simulink model "PID_simulation"  (Simulink 8.5)
settings: Solver=ode113  StartTime=0.0  StopTime=14  RelTol=1e-12  AbsTol=1e-12
undefined symbols (not defined in the file): P, sample_time
settings Model: Creator=Paul_local  LastModifiedBy=User
settings DataIOCC: SaveFormat=StructureWithTime  SignalLoggingSaveFormat=Dataset
settings OptimizationCC: ExpressionDepthLimit=128  EfficientFloat2IntCast=on
settings DebuggingCC: UnderspecifiedInitializationDetection=Simplified  MergeDetectMultiDrivingBlocksExec=error  FcnCallInpInsideContextMsg=EnableAllAsError  StateNameClashWarn=none
settings HardwareCC: ProdBitPerLong=64  ProdBitPerPointer=64  ProdLargestAtomicFloat=Float  ProdIntDivRoundTo=Zero  ProdEndianess=LittleEndian  ProdWordSize=64  ProdHWDeviceType=Intel->x86-64 (Windows64)
settings RTWCC: CheckMdlBeforeBuild=Warning
settings GRTTargetCC: GeneratePreprocessorConditionals=Use local settings  CombineOutputUpdateFcns=on  GRTInterface=off
settings ConfigComp: CovMetricSettings=dw  CovHtmlReporting=on  CovSaveCumulativeToWorkspaceVar=on  CovSaveSingleToWorkspaceVar=on  CovExternalEMLEnable=off

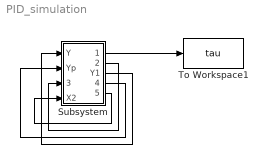
== system PID_simulation ==
  Subsystem : Subsystem
  To Workspace1 : ToWorkspace  VariableName=tau  SaveFormat=Structure With Time  SampleTime=-1
  wires:
  Subsystem/2(Ym1) -> Subsystem/3(Ym)
  Subsystem/5(x21) -> Subsystem/4(X2)
  Subsystem/3(Y1) -> Subsystem/1(Y)
  Subsystem/4(Yp1) -> Subsystem/2(Yp)
  Subsystem/1(tau) -> To Workspace1/1

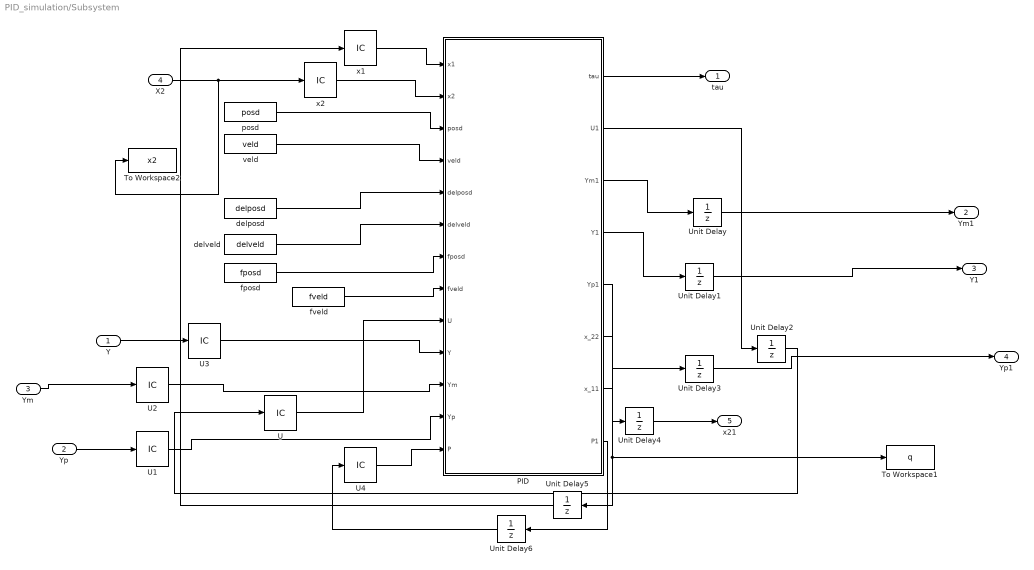
== system PID_simulation/Subsystem ==
  Y : Inport  PortDimensions=[14]
  Yp : Inport  Port=2  PortDimensions=[14]
  Ym : Inport  Port=3  PortDimensions=[14]
  X2 : Inport  Port=4  PortDimensions=[7]
  PID : MATLAB Function  TreatAsAtomicUnit=on
  To Workspace1 : ToWorkspace  VariableName=q  SaveFormat=Structure With Time  SampleTime=-1
  To Workspace2 : ToWorkspace  VariableName=x2  SaveFormat=Structure With Time  SampleTime=-1
  U : InitialCondition  Value=[0 0 0 0 0 0 0]
  U1 : InitialCondition  Value=[-0.1106,-1.9490,-0.0192,3.18400,0.2825,0.0969,-0.2798 0 0 0 0 0 0 0]
  U2 : InitialCondition  Value=[-0.1106,-1.9490,-0.0192,3.18400,0.2825,0.0969,-0.2798 0 0 0 0 0 0 0]
  U3 : InitialCondition  Value=[-0.1106,-1.9490,-0.0192,3.18400,0.2825,0.0969,-0.2798 0 0 0 0 0 0 0]
  U4 : InitialCondition  Value=P
  Unit Delay : UnitDelay  InitialCondition=[-0.1106,-1.9490,-0.0192,3.18400,0.2825,0.0969,-0.2798 0 0 0 0 0 0 0]  SampleTime=sample_time
  Unit Delay1 : UnitDelay  InitialCondition=[-0.1106,-1.9490,-0.0192,3.18400,0.2825,0.0969,-0.2798 0 0 0 0 0 0 0]  SampleTime=sample_time
  Unit Delay2 : UnitDelay  SampleTime=sample_time
  Unit Delay3 : UnitDelay  InitialCondition=[-0.1106,-1.9490,-0.0192,3.18400,0.2825,0.0969,-0.2798 0 0 0 0 0 0 0]  SampleTime=sample_time
  Unit Delay4 : UnitDelay  SampleTime=sample_time
  Unit Delay5 : UnitDelay  InitialCondition=[-0.1106,-1.9490,-0.0192,3.18400,0.2825,0.0969,-0.2798]  SampleTime=sample_time
  Unit Delay6 : UnitDelay  SampleTime=sample_time
  "delposd " : FromWorkspace  VariableName=delposd  SampleTime=sample_time
  delveld : FromWorkspace  VariableName=delveld  SampleTime=sample_time
  "fposd " : FromWorkspace  VariableName=fposd  SampleTime=sample_time
  fveld : FromWorkspace  VariableName=fveld  SampleTime=sample_time
  "posd " : FromWorkspace  VariableName=posd  SampleTime=sample_time
  veld : FromWorkspace  VariableName=veld  SampleTime=sample_time
  x1 : InitialCondition  Value=[-0.1106,-1.9490,-0.192,3.18400,0.2825,0.0969,-0.2798]
  x2 : InitialCondition  Value=[0 0 0 0 0 0 0]
  tau : Outport
  Ym1 : Outport  Port=2  PortDimensions=[14]
  Y1 : Outport  Port=3  PortDimensions=[14]
  Yp1 : Outport  Port=4  PortDimensions=[14]
  x21 : Outport  Port=5  PortDimensions=[7]
  wires:
  x1/1 -> PID/1(x1)
  PID/6(x_22) -> Unit Delay4/1
  "delposd "/1 -> PID/5(delposd)
  veld/1 -> PID/4(veld)
  delveld/1 -> PID/6(delveld)
  Y/1 -> U3/1
  x2/1 -> PID/2(x2)
  U3/1 -> PID/10(Y)
  Ym/1 -> U2/1
  Yp/1 -> U1/1
  "posd "/1 -> PID/3(posd)
  Unit Delay2/1 -> U/1
  PID/2(U1) -> Unit Delay2/1
  U/1 -> PID/9(U)
  U2/1 -> PID/11(Ym)
  PID/3(Ym1) -> Unit Delay/1
  fveld/1 -> PID/8(fveld)
  "fposd "/1 -> PID/7(fposd)
  Unit Delay/1 -> Ym1/1
  PID/7(x_11) -> Unit Delay5/1, To Workspace1/1
  PID/1(tau) -> tau/1
  U1/1 -> PID/12(Yp)
  X2/1 -> To Workspace2/1, x2/1
  PID/4(Y1) -> Unit Delay1/1
  Unit Delay1/1 -> Y1/1
  Unit Delay3/1 -> Yp1/1
  PID/5(Yp1) -> Unit Delay3/1
  Unit Delay5/1 -> x1/1
  Unit Delay4/1 -> x21/1
  U4/1 -> PID/13(P)
  PID/8(P1) -> Unit Delay6/1
  Unit Delay6/1 -> U4/1

== matlab function Subsystem/PID ==
  data: x1 input double; x2 input double; posd input double; tau output double; veld input double; delposd input double; delveld input double; fposd input double; fveld input double; U input double; U1 output double; Ym1 output double; Y1 output double; Yp1 output double; x_22 output double; Y input double; Ym input double; Yp input double; x_11 output double; P input double; P1 output double
%
% gravComp7DOFNum Compute inverse dynamics via recursive Newton-Euler formulation
%
% Recursive Newton-Euler for standard Denavit-Hartenberg notation.
%

% Copyright (C) 1993-2011, by Peter I. Corke
%
% This file originally was part of The Robotics Toolbox for Matlab (RTB).
%
% http://www.petercorke.com

%
% Simplified from rne_dh for 7DOF WAM to compute only torque from gravity by Hans Vorsteveld
% Does not use structures from RTB, only the RNE algorithm
%

function [tau,U1,Ym1,Y1,Yp1,x_22,x_11,P1] = PID(x1,x2,posd,veld,delposd,delveld,fposd,fveld,U,Y,Ym,Yp,P)

%-------------------------------------------------------------------------------------
%   SETUP THE ARM
%-------------------------------------------------------------------------------------    
    n = 14;p = 7; q = 14;
    
 Ts=0.002; 


 
 


yddel=[delposd;delveld];
yd = [posd;veld];
fyd=[fposd;fveld];


 

%initial conditions
%x1 = [-0.11060;-1.949;-0.1920;3.1840;0.2825;0.09690;-0.27980];
%x2 = zeros(7,1);
%U = zeros(7,1);
Ae = 0.9*eye(n);
C= eye(14);
Ce = C;
Iq = eye(q);
Oq = zeros(q);
H = [Iq Oq Oq -Ce*Ae;Iq Oq Oq zeros(q,n);Oq Iq Oq zeros(q,n);zeros(n,q) zeros(n,q) zeros(n,q) Ae];
Ib = zeros(3*q,3*q+n);
for k11 = 1:3*q,Ib(k11,k11) = 1;end
sig = 1e-3;
sigR = sig;
sigQ = 1e-4;%1e-3;
alfa = 1e0;
beta = 1e-2;
p1 = alfa*ones(1,3*q);
p2 = beta*ones(1,n);
pb = [p1 p2];

r1 = 5;
r2 = 50;
r3 = 1.5;
rv = 10;
rbb1 = r1*sig^2*ones(1,q/2);
rbb2 = r2*0.1*sig^2*ones(1,q/2);
rbb12 = [rbb1 rbb2];
rbb = [r3*rbb12 rbb12 rbb12];
 
Rb = 1*diag(rbb);
Q = 0*sigQ^2*eye(n);





 Be = Ts*[zeros(7,7);inv(D(x1))];
    Delyd=fyd-yd;
    Del2yd = Delyd*Delyd';
   
    Gd = [Del2yd Oq Oq zeros(q,n); Oq Oq Oq zeros(q,n); Oq Oq Oq zeros(q,n);zeros(n,q) zeros(n,q) zeros(n,q) Q];
   
    
    
   EE = [Ce*Be;zeros(q,p);zeros(q,p);-Be];
    K = inv(EE'*EE)*EE'*H*P*Ib'*inv(Ib*P*Ib' + Rb);
    PHI = H - EE*K*Ib;
    %if max(abs(eig(PHI))) > 1, disp('max(abs(eig(PHI))) > 1'),tk, pause(1),end
   
    P1 = PHI*P*PHI' + EE*K*Rb*K'*EE' + Gd;
    K1 = K(:,1:q);
    K2 = K(:,q+1:2*q);
    K3 = K(:,2*q+1:3*q);
    
    
      %  E = yd - Y ;
       % Ep = ydfut-Yp ;
        %U = U + K1*Ep + K2*E;
        %Ym = Y;
        %Y = Yp;
         %x_1 = x1 ;
       
         %x_11 = x_1; %Since at t=0, velocity is zero
        %XX2 = zeros(7,1);
        %x_22= (-inv(D(x_1))*(transpose(G(x_1)))+ inv(D(x_1))*U)*Ts + XX2 ;
        %Yp = [x_11' x_22']';
       
    
        Em = yddel - Ym ;
        E = yd - Y ;
        Ep = fyd-Yp ;
        U1 = U + K1*Ep + K2*E + K3*Em;
        Ym1 = Y;
        Y1 = Yp;
        
       
        
        
         
       Ts=0.002;   
        % In experimental work you do not add noise instead you only use measurement of position
        x_11 =  x2*Ts + x1; % Here we are estimating position using the extimate of x2 and measurement of x1 at present time
        
        %XX2 = (x_11-x_1)/Ts; 
        %XX2 = (x1-x1d)/Ts; 
        
        %x_22= (-inv(D(pos_meas))*((G(pos_meas)))+ inv(D(pos_meas))*U)*Ts + XX2 ;
        x3=(-inv(D(x1))*((G(x1)))+ inv(D(x1))*U1);
       x_22=  x2 + Ts*x3;
        
        Yp1 = [x_11' x_22']';
       
        tau=U1;
        
        
        
        
        
    
   
end 

function G = G(q)

DH_a = [0 0 0.045 -0.045 0 0 0];
    DH_d = [0 0 .55 0 0.3 0 0.061];
    DH_alpha = [-pi/2 pi/2 -pi/2 pi/2 -pi/2 pi/2 0];
 
    m = [10.7676 3.87 1.8022 2.4 0.1237 0.4979886 0.07548270];
    
    com = zeros(3,7);
    com(:,1) = [-0.00443422; 0.12189039; -0.00066489];
    com(:,2) = [-0.00236983; 0.03105614; 0.01542114 ];
    com(:,3) = [-0.03825858; 0.20750770; 0.00003309];
    com(:,4) = [ 0.00498512;-0.00022942;0.13271662 ];
    com(:,5) = [0.00008921;0.00511217;0.00435824];
    com(:,6) = [-0.00012262;-0.01703194;0.02468336];
    com(:,7) = [-0.00007974;0.00016313;-0.00323552 ];
     
    
    T = zeros(4,4,7);
     
for j=1:7,
        a = DH_a(j);
        d = DH_d(j);
        alpha = DH_alpha(j);
        T(:,:,j) = getTransformDH(a, d, alpha, q(j));
end 
comstar = zeros(4,7);
    comstar(:,1) = [com(:,1);1];
    comstar(:,2) = [com(:,2);1];
    comstar(:,3) = [com(:,3);1];
    comstar(:,4) = [com(:,4);1];
    comstar(:,5) = [com(:,5);1];
    comstar(:,6) = [com(:,6);1];
    comstar(:,7) = [ com(:,7);1];
  
    Q=[0,-1,0,0;
     1,0,0,0;
     0,0,0,0;
     0,0,0,0];
   
 gravity=[0,0,-9.81,0];
 G=zeros(7,1);
 
   G(1)= -m(1)*gravity*Q*T(:,:,1)*comstar(:,1)-m(2)*gravity*Q*T(:,:,1)*T(:,:,2)*comstar(:,2)-m(3)*gravity*Q*T(:,:,1)*T(:,:,2)*T(:,:,3)*comstar(:,3)-m(4)*gravity*Q*T(:,:,1)*T(:,:,2)*T(:,:,3)*T(:,:,4)*comstar(:,4)-m(5)*gravity*Q*T(:,:,1)*T(:,:,2)*T(:,:,3)*T(:,:,4)*T(:,:,5)*comstar(:,5)-m(6)*gravity*Q*T(:,:,1)*T(:,:,2)*T(:,:,3)*T(:,:,4)*T(:,:,5)*T(:,:,6)*comstar(:,6)-m(7)*gravity*Q*T(:,:,1)*T(:,:,2)*T(:,:,3)*T(:,:,4)*T(:,:,5)*T(:,:,6)*T(:,:,7)*comstar(:,7);   
   G(2)= -m(2)*gravity*T(:,:,1)*Q*T(:,:,2)*comstar(:,2)-m(3)*gravity*T(:,:,1)*Q*T(:,:,2)*T(:,:,3)*comstar(:,3)-m(4)*gravity*T(:,:,1)*Q*T(:,:,2)*T(:,:,3)*T(:,:,4)*comstar(:,4)-m(5)*gravity*T(:,:,1)*Q*T(:,:,2)*T(:,:,3)*T(:,:,4)*T(:,:,5)*comstar(:,5)-m(6)*gravity*T(:,:,1)*Q*T(:,:,2)*T(:,:,3)*T(:,:,4)*T(:,:,5)*T(:,:,6)*comstar(:,6)-m(7)*gravity*T(:,:,1)*Q*T(:,:,2)*T(:,:,3)*T(:,:,4)*T(:,:,5)*T(:,:,6)*T(:,:,7)*comstar(:,7);
   G(3)= -m(3)*gravity*T(:,:,1)*T(:,:,2)*Q*T(:,:,3)*comstar(:,3)-m(4)*gravity*T(:,:,1)*T(:,:,2)*Q*T(:,:,3)*T(:,:,4)*comstar(:,4)-m(5)*gravity*T(:,:,1)*T(:,:,2)*Q*T(:,:,3)*T(:,:,4)*T(:,:,5)*comstar(:,5)-m(6)*gravity*T(:,:,1)*T(:,:,2)*Q*T(:,:,3)*T(:,:,4)*T(:,:,5)*T(:,:,6)*comstar(:,6)-m(7)*gravity*T(:,:,1)*T(:,:,2)*Q*T(:,:,3)*T(:,:,4)*T(:,:,5)*T(:,:,6)*T(:,:,7)*comstar(:,7);
   G(4)= -m(4)*gravity*T(:,:,1)*T(:,:,2)*T(:,:,3)*Q*T(:,:,4)*comstar(:,4)-m(5)*gravity*T(:,:,1)*T(:,:,2)*T(:,:,3)*Q*T(:,:,4)*T(:,:,5)*comstar(:,5)-m(6)*gravity*T(:,:,1)*T(:,:,2)*T(:,:,3)*Q*T(:,:,4)*T(:,:,5)*T(:,:,6)*comstar(:,6)-m(7)*gravity*T(:,:,1)*T(:,:,2)*T(:,:,3)*Q*T(:,:,4)*T(:,:,5)*T(:,:,6)*T(:,:,7)*comstar(:,7);
   G(5)= -m(5)*gravity*T(:,:,1)*T(:,:,2)*T(:,:,3)*T(:,:,4)*Q*T(:,:,5)*comstar(:,5)-m(6)*gravity*T(:,:,1)*T(:,:,2)*T(:,:,3)*T(:,:,4)*Q*T(:,:,5)*T(:,:,6)*comstar(:,6)-m(7)*gravity*T(:,:,1)*T(:,:,2)*T(:,:,3)*T(:,:,4)*Q*T(:,:,5)*T(:,:,6)*T(:,:,7)*comstar(:,7);
   G(6)= -m(6)*gravity*T(:,:,1)*T(:,:,2)*T(:,:,3)*T(:,:,4)*T(:,:,5)*Q*T(:,:,6)*comstar(:,6)-m(7)*gravity*T(:,:,1)*T(:,:,2)*T(:,:,3)*T(:,:,4)*T(:,:,5)*Q*T(:,:,6)*T(:,:,7)*comstar(:,7);
   G(7)= -m(7)*gravity*T(:,:,1)*T(:,:,2)*T(:,:,3)*T(:,:,4)*T(:,:,5)*T(:,:,6)*Q*T(:,:,7)*comstar(:,7);
   
end 
function bq = bq(qd)
 
 
 
s=20;
bc = [2.516; 2.581; 2.038; 0.956; 0.323; 0.315; 0.066];
B =  [1.142; 0.946; 0.309; 0.255; 0.025; 0.039; 0.004];
 
bq = bc.*atan(s*qd)*2/pi+B.*qd;
end 

function D =D(q)
DH_a = [0 0 0.045 -0.045 0 0 0];
    DH_d = [0 0 .55 0 0.3 0 0.061];
    DH_alpha = [-pi/2 pi/2 -pi/2 pi/2 -pi/2 pi/2 0];
 
    m = [10.7676 3.87 1.8022 2.4 0.1237 0.4179886 0.07548270];
    
     
    
    com = zeros(3,7);
   com(:,1) = [-0.00443422; 0.12189039; -0.00066489];
    com(:,2) = [-0.00236983; 0.03105614; 0.01542114 ];
    com(:,3) = [-0.03825858; 0.20750770; 0.00003309];
    com(:,4) = [ 0.00498512;-0.00022942;0.13271662 ];
    com(:,5) = [0.00008921;0.00511217;0.00435824];
    com(:,6) = [-0.00012262;-0.01703194;0.02468336];
    com(:,7) = [-0.00007974;0.00016313;-0.00323552 ];
     
    I=zeros(3,3,7);
    
     I(:,:,1) = [ 0.29486350 , -0.00795023 ,-0.00009311;
                 -0.00795023 , 0.11350017 , -0.00018711;
                -0.00009311 , -0.00018711 , 0.25065343];
    I(:,:,2) =[0.02606840 ,-0.00001346 , -0.00011701;
               -0.00001346,  0.01472202 ,0.00003659;
               -0.00011701 , 0.00003659,  0.01934814];
    I(:,:,3) = [0.13671601,  -0.01680434,  0.00000510;
               -0.01680434 , 0.00588354 , -0.00000530;
                0.00000510 , -0.00000530 , 0.13951371];
    I(:,:,4) = [ 0.05719268 , 0.00001467 , 0.00008193;
                 0.00001467 , 0.05716470 , -0.00009417;
                 0.00008193 , -0.00009417 , 0.00300441] ;
    I(:,:,5) =[0.00005587 , 0.00000026,  0.00000000;
               0.00000026 , 0.00007817,  -0.00000083;
               0.00000000 , -0.00000083,  0.00006594];
    I(:,:,6) = [0.00093106,  0.00000148 , -0.00000201;
                0.00000148,  0.00049833 , -0.00022162;
               -0.00000201,  -0.00022162,  0.00057483];
   I(:,:,7) = [0.00003845,  -0.00000019 , 0.00000002;
                -0.00000019, 0.00003878 , -0.00000004;
                0.00000002 ,  -0.00000004, 0.00007408 ];
            T=zeros(4,4,7);
  
             
for j=1:7,
        a = DH_a(j);
        d = DH_d(j);
        alpha = DH_alpha(j);
        T(:,:,j) = getTransformDH(a, d, alpha, q(j));
end 
 
 
 
 
   comstar = zeros(4,7);
    comstar(:,1) = [com(:,1);1];
    comstar(:,2) = [com(:,2);1];
    comstar(:,3) = [com(:,3);1];
    comstar(:,4) = [com(:,4);1];
    comstar(:,5) = [com(:,5);1];
    comstar(:,6) = [com(:,6);1];
    comstar(:,7) = [ com(:,7);1];
  
    Q=[0,-1,0,0;
     1,0,0,0;
     0,0,0,0;
     0,0,0,0];
   
U=zeros(4,4,7,7);
   U(:,:,1,1)= Q*T(:,:,1);
   U(:,:,2,1)= Q*T(:,:,1)*T(:,:,2);
   U(:,:,3,1)= Q*T(:,:,1)*T(:,:,2)*T(:,:,3);
   U(:,:,4,1)= Q*T(:,:,1)*T(:,:,2)*T(:,:,3)*T(:,:,4);
   U(:,:,5,1)= Q*T(:,:,1)*T(:,:,2)*T(:,:,3)*T(:,:,4)*T(:,:,5);
   U(:,:,6,1)= Q*T(:,:,1)*T(:,:,2)*T(:,:,3)*T(:,:,4)*T(:,:,5)*T(:,:,6);
   U(:,:,7,1)= Q*T(:,:,1)*T(:,:,2)*T(:,:,3)*T(:,:,4)*T(:,:,5)*T(:,:,6)*T(:,:,7);
   
   
   U(:,:,2,2)= T(:,:,1)*Q*T(:,:,2);
   U(:,:,3,2)= T(:,:,1)*Q*T(:,:,2)*T(:,:,3);
   U(:,:,4,2)= T(:,:,1)*Q*T(:,:,2)*T(:,:,3)*T(:,:,4);
   U(:,:,5,2)= T(:,:,1)*Q*T(:,:,2)*T(:,:,3)*T(:,:,4)*T(:,:,5);
   U(:,:,6,2)= T(:,:,1)*Q*T(:,:,2)*T(:,:,3)*T(:,:,4)*T(:,:,5)*T(:,:,6);
   U(:,:,7,2)= T(:,:,1)*Q*T(:,:,2)*T(:,:,3)*T(:,:,4)*T(:,:,5)*T(:,:,6)*T(:,:,7);
   
  
   U(:,:,3,3)= T(:,:,1)*T(:,:,2)*Q*T(:,:,3);
   U(:,:,4,3)= T(:,:,1)*T(:,:,2)*Q*T(:,:,3)*T(:,:,4);
   U(:,:,5,3)= T(:,:,1)*T(:,:,2)*Q*T(:,:,3)*T(:,:,4)*T(:,:,5);
   U(:,:,6,3)= T(:,:,1)*T(:,:,2)*Q*T(:,:,3)*T(:,:,4)*T(:,:,5)*T(:,:,6);
   U(:,:,7,3)= T(:,:,1)*T(:,:,2)*Q*T(:,:,3)*T(:,:,4)*T(:,:,5)*T(:,:,6)*T(:,:,7);
   
   U(:,:,4,4)= T(:,:,1)*T(:,:,2)*T(:,:,3)*Q*T(:,:,4);
   U(:,:,5,4)= T(:,:,1)*T(:,:,2)*T(:,:,3)*Q*T(:,:,4)*T(:,:,5);
   U(:,:,6,4)= T(:,:,1)*T(:,:,2)*T(:,:,3)*Q*T(:,:,4)*T(:,:,5)*T(:,:,6);
   U(:,:,7,4)= T(:,:,1)*T(:,:,2)*T(:,:,3)*Q*T(:,:,4)*T(:,:,5)*T(:,:,6)*T(:,:,7);
   
   U(:,:,5,5)= T(:,:,1)*T(:,:,2)*T(:,:,3)*T(:,:,4)*Q*T(:,:,5);
   U(:,:,6,5)= T(:,:,1)*T(:,:,2)*T(:,:,3)*T(:,:,4)*Q*T(:,:,5)*T(:,:,6);
   U(:,:,7,5)= T(:,:,1)*T(:,:,2)*T(:,:,3)*T(:,:,4)*Q*T(:,:,5)*T(:,:,6)*T(:,:,7);
   
   U(:,:,6,6)= T(:,:,1)*T(:,:,2)*T(:,:,3)*T(:,:,4)*T(:,:,5)*Q*T(:,:,6);
   U(:,:,7,6)= T(:,:,1)*T(:,:,2)*T(:,:,3)*T(:,:,4)*T(:,:,5)*Q*T(:,:,6)*T(:,:,7);
   
   U(:,:,7,7)= T(:,:,1)*T(:,:,2)*T(:,:,3)*T(:,:,4)*T(:,:,5)*T(:,:,6)*Q*T(:,:,7);
   
   
   
  
   J=zeros(4,4,7);
 
   
   J(:,:,1)=[0.5*(-I(1,1,1)+I(2,2,1)+I(3,3,1)), I(1,2,1), I(1,3,1), m(1)*com(1,1);
             I(1,2,1) ,0.5*(I(1,1,1)-I(2,2,1)+I(3,3,1)), I(2,3,1), m(1)*com(2,1);
             I(1,3,1), I(2,3,1), 0.5*(I(1,1,1)+I(2,2,1)-I(3,3,1)), m(1)*com(3,1);
              m(1)*com(1,1), m(1)*com(2,1), m(1)*com(3,1), m(1)];
   
    J(:,:,2)=[0.5*(-I(1,1,2)+I(2,2,2)+I(3,3,2)), I(1,2,2), I(1,3,2), m(2)*com(1,2);
             I(1,2,2) ,0.5*(I(1,1,2)-I(2,2,2)+I(3,3,2)), I(2,3,2), m(2)*com(2,2);
             I(1,3,2), I(2,3,2), 0.5*(I(1,1,2)+I(2,2,2)-I(3,3,2)), m(2)*com(3,2);
              m(2)*com(1,2), m(2)*com(2,2), m(2)*com(3,2), m(2)];
   
          
     J(:,:,3)=[0.5*(-I(1,1,3)+I(2,2,3)+I(3,3,3)), I(1,2,3), I(1,3,3), m(3)*com(1,3);
             I(1,2,3) ,0.5*(I(1,1,3)-I(2,2,3)+I(3,3,3)), I(2,3,3), m(3)*com(2,3);
             I(1,3,3), I(2,3,3), 0.5*(I(1,1,3)+I(2,2,3)-I(3,3,3)), m(3)*com(3,3);
              m(3)*com(1,3), m(3)*com(2,3), m(3)*com(3,3), m(3)];      
   
   
    J(:,:,4)=[0.5*(-I(1,1,4)+I(2,2,4)+I(3,3,4)), I(1,2,4), I(1,3,4), m(4)*com(1,4);
             I(1,2,4) ,0.5*(I(1,1,4)-I(2,2,4)+I(3,3,4)), I(2,3,4), m(4)*com(2,4);
             I(1,3,4), I(2,3,4), 0.5*(I(1,1,4)+I(2,2,4)-I(3,3,4)), m(4)*com(3,4);
              m(4)*com(1,4), m(4)*com(2,4), m(4)*com(3,4), m(4)];
   
   
    J(:,:,5)=[0.5*(-I(1,1,5)+I(2,2,5)+I(3,3,5)), I(1,2,5), I(1,3,5), m(5)*com(1,5);
             I(1,2,5) ,0.5*(I(1,1,5)-I(2,2,5)+I(3,3,5)), I(2,3,5), m(5)*com(2,5);
             I(1,3,5), I(2,3,5), 0.5*(I(1,1,5)+I(2,2,5)-I(3,3,5)), m(5)*com(3,5);
              m(5)*com(1,5), m(5)*com(2,5), m(5)*com(3,5), m(5)];
   
   
    J(:,:,6)=[0.5*(-I(1,1,6)+I(2,2,6)+I(3,3,6)), I(1,2,6), I(1,3,6), m(6)*com(1,6);
             I(1,2,6) ,0.5*(I(1,1,6)-I(2,2,6)+I(3,3,6)), I(2,3,6), m(6)*com(2,6);
             I(1,3,6), I(2,3,6), 0.5*(I(1,1,6)+I(2,2,6)-I(3,3,6)), m(6)*com(3,6);
              m(6)*com(1,6), m(6)*com(2,6), m(6)*com(3,6), m(6)];
   
   
    J(:,:,7)=[0.5*(-I(1,1,7)+I(2,2,7)+I(3,3,7)), I(1,2,7), I(1,3,7), m(7)*com(1,7);
             I(1,2,7) ,0.5*(I(1,1,7)-I(2,2,7)+I(3,3,7)), I(2,3,7), m(7)*com(2,7);
             I(1,3,7), I(2,3,7), 0.5*(I(1,1,7)+I(2,2,7)-I(3,3,7)), m(7)*com(3,7);
              m(7)*com(1,7), m(7)*com(2,7), m(7)*com(3,7), m(7)];
   
   D=zeros(7,7);
    D(1,1)= trace(U(:,:,1,1)*J(:,:,1)*transpose(U(:,:,1,1))) + trace(U(:,:,2,1)*J(:,:,2)*transpose(U(:,:,2,1))) + trace(U(:,:,3,1)*J(:,:,3)*transpose(U(:,:,3,1))) + trace(U(:,:,4,1)*J(:,:,4)*transpose(U(:,:,4,1))) + trace(U(:,:,5,1)*J(:,:,5)*transpose(U(:,:,5,1))) + trace(U(:,:,6,1)*J(:,:,6)*transpose(U(:,:,6,1))) + trace(U(:,:,7,1)*J(:,:,7)*transpose(U(:,:,7,1))) ;
    D(1,2)= trace(U(:,:,2,2)*J(:,:,2)*transpose(U(:,:,2,1))) + trace(U(:,:,3,2)*J(:,:,3)*transpose(U(:,:,3,1))) + trace(U(:,:,4,2)*J(:,:,4)*transpose(U(:,:,4,1))) +trace(U(:,:,5,2)*J(:,:,5)*transpose(U(:,:,5,1))) + trace(U(:,:,6,2)*J(:,:,6)*transpose(U(:,:,6,1))) + trace(U(:,:,7,2)*J(:,:,7)*transpose(U(:,:,7,1))); 
    D(1,3)= trace(U(:,:,3,3)*J(:,:,3)*transpose(U(:,:,3,1)))+ trace(U(:,:,4,3)*J(:,:,4)*transpose(U(:,:,4,1)))+ trace(U(:,:,5,3)*J(:,:,5)*transpose(U(:,:,5,1)))+ trace(U(:,:,6,3)*J(:,:,6)*transpose(U(:,:,6,1)))+ trace(U(:,:,7,3)*J(:,:,7)*transpose(U(:,:,7,1))); 
    D(1,4)= trace(U(:,:,4,4)*J(:,:,4)*transpose(U(:,:,4,1)))+ trace(U(:,:,5,4)*J(:,:,5)*transpose(U(:,:,5,1)))+ trace(U(:,:,6,4)*J(:,:,6)*transpose(U(:,:,6,1)))+ trace(U(:,:,7,4)*J(:,:,7)*transpose(U(:,:,7,1)));
    D(1,5)= trace(U(:,:,5,5)*J(:,:,5)*transpose(U(:,:,5,1)))+ trace(U(:,:,6,5)*J(:,:,6)*transpose(U(:,:,6,1)))+ trace(U(:,:,7,5)*J(:,:,7)*transpose(U(:,:,7,1)));
    D(1,6)= trace(U(:,:,6,6)*J(:,:,6)*transpose(U(:,:,6,1)))+ trace(U(:,:,7,6)*J(:,:,7)*transpose(U(:,:,7,1)));
    D(1,7)= trace(U(:,:,7,7)*J(:,:,7)*transpose(U(:,:,7,1)));
    
    D(2,1)= trace(U(:,:,2,1)*J(:,:,2)*transpose(U(:,:,2,2)))+ trace(U(:,:,3,1)*J(:,:,3)*transpose(U(:,:,3,2)))+ trace(U(:,:,4,1)*J(:,:,4)*transpose(U(:,:,4,2)))+ trace(U(:,:,5,1)*J(:,:,5)*transpose(U(:,:,5,2)))+ trace(U(:,:,6,1)*J(:,:,6)*transpose(U(:,:,6,2)))+ trace(U(:,:,7,1)*J(:,:,7)*transpose(U(:,:,7,2)));
    D(2,2)= trace(U(:,:,2,2)*J(:,:,2)*transpose(U(:,:,2,2)))+ trace(U(:,:,3,2)*J(:,:,3)*transpose(U(:,:,3,2)))+ trace(U(:,:,4,2)*J(:,:,4)*transpose(U(:,:,4,2)))+ trace(U(:,:,5,2)*J(:,:,5)*transpose(U(:,:,5,2)))+ trace(U(:,:,6,2)*J(:,:,6)*transpose(U(:,:,6,2)))+ trace(U(:,:,7,2)*J(:,:,7)*transpose(U(:,:,7,2)));
    D(2,3)= trace(U(:,:,3,3)*J(:,:,3)*transpose(U(:,:,3,2)))+ trace(U(:,:,4,3)*J(:,:,4)*transpose(U(:,:,4,2)))+ trace(U(:,:,5,3)*J(:,:,5)*transpose(U(:,:,5,2)))+ trace(U(:,:,6,3)*J(:,:,6)*transpose(U(:,:,6,2)))+ trace(U(:,:,7,3)*J(:,:,7)*transpose(U(:,:,7,2))); 
    D(2,4)= trace(U(:,:,4,4)*J(:,:,4)*transpose(U(:,:,4,2)))+ trace(U(:,:,5,4)*J(:,:,5)*transpose(U(:,:,5,2)))+ trace(U(:,:,6,4)*J(:,:,6)*transpose(U(:,:,6,2)))+ trace(U(:,:,7,4)*J(:,:,7)*transpose(U(:,:,7,2))); 
    D(2,5)= trace(U(:,:,5,5)*J(:,:,5)*transpose(U(:,:,5,2)))+ trace(U(:,:,6,5)*J(:,:,6)*transpose(U(:,:,6,2)))+ trace(U(:,:,7,5)*J(:,:,7)*transpose(U(:,:,7,2)));
    D(2,6)= trace(U(:,:,6,6)*J(:,:,6)*transpose(U(:,:,6,2)))+ trace(U(:,:,7,6)*J(:,:,7)*transpose(U(:,:,7,2))); 
    D(2,7)= trace(U(:,:,7,7)*J(:,:,7)*transpose(U(:,:,7,2)));
  
    D(3,1)= trace(U(:,:,3,1)*J(:,:,3)*transpose(U(:,:,3,3)))+ trace(U(:,:,4,1)*J(:,:,4)*transpose(U(:,:,4,3)))+ trace(U(:,:,5,1)*J(:,:,5)*transpose(U(:,:,5,3)))+ trace(U(:,:,6,1)*J(:,:,6)*transpose(U(:,:,6,3)))+ trace(U(:,:,7,1)*J(:,:,7)*transpose(U(:,:,7,3)));
    D(3,2)= trace(U(:,:,3,2)*J(:,:,3)*transpose(U(:,:,3,3)))+ trace(U(:,:,4,2)*J(:,:,4)*transpose(U(:,:,4,3)))+ trace(U(:,:,5,2)*J(:,:,5)*transpose(U(:,:,5,3)))+ trace(U(:,:,6,2)*J(:,:,6)*transpose(U(:,:,6,3)))+ trace(U(:,:,7,2)*J(:,:,7)*transpose(U(:,:,7,3)));
    D(3,3)= trace(U(:,:,3,3)*J(:,:,3)*transpose(U(:,:,3,3)))+ trace(U(:,:,4,3)*J(:,:,4)*transpose(U(:,:,4,3)))+ trace(U(:,:,5,3)*J(:,:,5)*transpose(U(:,:,5,3)))+ trace(U(:,:,6,3)*J(:,:,6)*transpose(U(:,:,6,3)))+ trace(U(:,:,7,3)*J(:,:,7)*transpose(U(:,:,7,3)));
    D(3,4)= trace(U(:,:,4,4)*J(:,:,4)*transpose(U(:,:,4,3)))+ trace(U(:,:,5,4)*J(:,:,5)*transpose(U(:,:,5,3)))+ trace(U(:,:,6,4)*J(:,:,6)*transpose(U(:,:,6,3)))+ trace(U(:,:,7,4)*J(:,:,7)*transpose(U(:,:,7,3)));
    D(3,5)= trace(U(:,:,5,5)*J(:,:,5)*transpose(U(:,:,5,3)))+ trace(U(:,:,6,5)*J(:,:,6)*transpose(U(:,:,6,3)))+ trace(U(:,:,7,5)*J(:,:,7)*transpose(U(:,:,7,3)));
    D(3,6)= trace(U(:,:,6,6)*J(:,:,6)*transpose(U(:,:,6,3)))+ trace(U(:,:,7,6)*J(:,:,7)*transpose(U(:,:,7,3)));
    D(3,7)= trace(U(:,:,7,7)*J(:,:,7)*transpose(U(:,:,7,3)));
     
     
    D(4,1)= trace(U(:,:,4,1)*J(:,:,4)*transpose(U(:,:,4,4)))+ trace(U(:,:,5,1)*J(:,:,5)*transpose(U(:,:,5,4)))+ trace(U(:,:,6,1)*J(:,:,6)*transpose(U(:,:,6,4)))+ trace(U(:,:,7,1)*J(:,:,7)*transpose(U(:,:,7,4))); 
    D(4,2)= trace(U(:,:,4,2)*J(:,:,4)*transpose(U(:,:,4,4)))+ trace(U(:,:,5,2)*J(:,:,5)*transpose(U(:,:,5,4)))+ trace(U(:,:,6,2)*J(:,:,6)*transpose(U(:,:,6,4)))+ trace(U(:,:,7,2)*J(:,:,7)*transpose(U(:,:,7,4))); 
    D(4,3)= trace(U(:,:,4,3)*J(:,:,4)*transpose(U(:,:,4,4)))+ trace(U(:,:,5,3)*J(:,:,5)*transpose(U(:,:,5,4)))+ trace(U(:,:,6,3)*J(:,:,6)*transpose(U(:,:,6,4)))+ trace(U(:,:,7,3)*J(:,:,7)*transpose(U(:,:,7,4)));
    D(4,4)= trace(U(:,:,4,4)*J(:,:,4)*transpose(U(:,:,4,4)))+ trace(U(:,:,5,4)*J(:,:,5)*transpose(U(:,:,5,4)))+ trace(U(:,:,6,4)*J(:,:,6)*transpose(U(:,:,6,4)))+ trace(U(:,:,7,4)*J(:,:,7)*transpose(U(:,:,7,4)));
    D(4,5)= trace(U(:,:,5,5)*J(:,:,5)*transpose(U(:,:,5,4)))+ trace(U(:,:,6,5)*J(:,:,6)*transpose(U(:,:,6,4)))+ trace(U(:,:,7,5)*J(:,:,7)*transpose(U(:,:,7,4)));
    D(4,6)= trace(U(:,:,6,6)*J(:,:,6)*transpose(U(:,:,6,4)))+ trace(U(:,:,7,6)*J(:,:,7)*transpose(U(:,:,7,4))); 
    D(4,7)= trace(U(:,:,7,7)*J(:,:,7)*transpose(U(:,:,7,4)));
    
    D(5,1)= trace(U(:,:,5,1)*J(:,:,5)*transpose(U(:,:,5,5)))+ trace(U(:,:,6,1)*J(:,:,6)*transpose(U(:,:,6,5)))+ trace(U(:,:,7,1)*J(:,:,7)*transpose(U(:,:,7,5)));
    D(5,2)= trace(U(:,:,5,2)*J(:,:,5)*transpose(U(:,:,5,5)))+ trace(U(:,:,6,2)*J(:,:,6)*transpose(U(:,:,6,5)))+ trace(U(:,:,7,2)*J(:,:,7)*transpose(U(:,:,7,5)));
    D(5,3)= trace(U(:,:,5,3)*J(:,:,5)*transpose(U(:,:,5,5)))+ trace(U(:,:,6,3)*J(:,:,6)*transpose(U(:,:,6,5)))+ trace(U(:,:,7,3)*J(:,:,7)*transpose(U(:,:,7,5))); 
    D(5,4)= trace(U(:,:,5,4)*J(:,:,5)*transpose(U(:,:,5,5)))+ trace(U(:,:,6,4)*J(:,:,6)*transpose(U(:,:,6,5)))+ trace(U(:,:,7,4)*J(:,:,7)*transpose(U(:,:,7,5))); 
    D(5,5)= trace(U(:,:,5,5)*J(:,:,5)*transpose(U(:,:,5,5)))+ trace(U(:,:,6,5)*J(:,:,6)*transpose(U(:,:,6,5)))+ trace(U(:,:,7,5)*J(:,:,7)*transpose(U(:,:,7,5)));
    D(5,6)= trace(U(:,:,6,6)*J(:,:,6)*transpose(U(:,:,6,5)))+ trace(U(:,:,7,6)*J(:,:,7)*transpose(U(:,:,7,5))); 
    D(5,7)= trace(U(:,:,7,7)*J(:,:,7)*transpose(U(:,:,7,5)));
    
    D(6,1)= trace(U(:,:,6,1)*J(:,:,6)*transpose(U(:,:,6,6)))+ trace(U(:,:,7,1)*J(:,:,7)*transpose(U(:,:,7,6)));
    D(6,2)= trace(U(:,:,6,2)*J(:,:,6)*transpose(U(:,:,6,6)))+ trace(U(:,:,7,2)*J(:,:,7)*transpose(U(:,:,7,6)));
    D(6,3)= trace(U(:,:,6,3)*J(:,:,6)*transpose(U(:,:,6,6)))+ trace(U(:,:,7,3)*J(:,:,7)*transpose(U(:,:,7,6))); 
    D(6,4)= trace(U(:,:,6,4)*J(:,:,6)*transpose(U(:,:,6,6)))+ trace(U(:,:,7,4)*J(:,:,7)*transpose(U(:,:,7,6))); 
    D(6,5)= trace(U(:,:,6,5)*J(:,:,6)*transpose(U(:,:,6,6)))+ trace(U(:,:,7,5)*J(:,:,7)*transpose(U(:,:,7,6))); 
    D(6,6)= trace(U(:,:,6,6)*J(:,:,6)*transpose(U(:,:,6,6)))+ trace(U(:,:,7,6)*J(:,:,7)*transpose(U(:,:,7,6))); 
    D(6,7)= trace(U(:,:,7,7)*J(:,:,7)*transpose(U(:,:,7,6)));
    
    D(7,1)= trace(U(:,:,7,1)*J(:,:,7)*transpose(U(:,:,7,7)));
    D(7,2)= trace(U(:,:,7,2)*J(:,:,7)*transpose(U(:,:,7,7)));
    D(7,3)= trace(U(:,:,7,3)*J(:,:,7)*transpose(U(:,:,7,7)));
    D(7,4)= trace(U(:,:,7,4)*J(:,:,7)*transpose(U(:,:,7,7)));
    D(7,5)= trace(U(:,:,7,5)*J(:,:,7)*transpose(U(:,:,7,7)));
    D(7,6)= trace(U(:,:,7,6)*J(:,:,7)*transpose(U(:,:,7,7)));
    D(7,7)= trace(U(:,:,7,7)*J(:,:,7)*transpose(U(:,:,7,7)));
end 



function T = getTransformDH(a,d,alpha,q)
    ct = cos(q);
    st = sin(q);
    cb = cos(alpha);
    sb = sin(alpha);
    
    T = [ ct, -st*cb,  st*sb, a*ct;
          st,  ct*cb, -ct*sb, a*st;
          0, sb, cb, d;
          0, 0, 0, 1 ];
end
